simulink model "TestTransitionTypeHandler"  (R2016b)
settings: Solver=FixedStepAuto  StartTime=0.0  StopTime=10.0  FixedStep=0.002  RelTol=1e-3  EnableMultiTasking=on
undefined symbols (not defined in the file): ControlStrategy
libraries: slrtlib x1
settings Model: SimulationMode=external  Creator=march  LastModifiedBy=march
settings SolverCC: EnableConcurrentExecution=on
settings DataIOCC: SaveFormat=StructureWithTime
settings OptimizationCC: BlockReduction=off  OptimizeBlockIOStorage=off  BufferReuse=off  GlobalBufferReuse=off  ExpressionFolding=off  LocalBlockOutputs=off
settings HardwareCC: ProdBitPerPointer=32  ProdBitPerSizeT=32  ProdBitPerPtrDiffT=32  ProdLargestAtomicFloat=None  ProdWordSize=32  ProdLongLongMode=on  ProdHWDeviceType=Generic->32-bit x86 compatible
settings RTWCC: SystemTargetFile=slrt.tlc  TemplateMakefile=slrt_default_tmf  Description=Simulink Real-Time  RTWCompilerOptimization=on

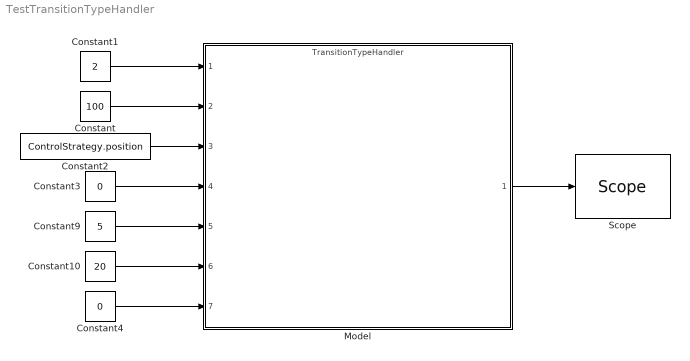
== system TestTransitionTypeHandler ==
  Constant : Constant  Value=100
  Constant1 : Constant  Value=2
  Constant10 : Constant  Value=20
  Constant2 : Constant  Value=ControlStrategy.position
  Constant3 : Constant  Value=0
  Constant4 : Constant  Value=0
  Constant9 : Constant  Value=5
  Model : ModelReference  ModelNameDialog=TransitionTypeHandler  SimulationMode=Normal  ModelReferenceVersion=1.17
  "Scope " : slrtlib/Displays and Logging/Scope   scopeno=1  scopetype=Target  autostart=on  viewmode=Graphical rolling  formatstr='%15.6f'  grid=on  ylimits=[-100,100]  nosamples=2500  noprepostsamples=0  interleave=1  triggermode=FreeRun  triggersignal=1  trigsignalfromport=off  triggerlevel=0.0  triggerslope=Either  triggerscope=1  triggersample=0  filename=data.dat  mode=Lazy  writesize=512  autorestart=off  dynamicfilemode=off  maxwritefilesize=512*1024^2
  wires:
  Constant1/1 -> Model/1
  Constant/1 -> Model/2
  Constant2/1 -> Model/3
  Constant3/1 -> Model/4
  Constant4/1 -> Model/7
  Constant9/1 -> Model/5
  Constant10/1 -> Model/6
  Model/1 -> "Scope "/1
